simulink model "Elektromagnet_Simscape_Integrated_Model"  (R2025a)
settings: Solver=VariableStepAuto  StartTime=0.0  StopTime=T_sim  RelTol=1e-3
PreLoadFcn:
  | init_simscape_simulation
InitFcn:
  | %init_simscape_simulation
values from neighbouring files (symbols this model uses):
  T_sim = 0.2    [init_simscape_simulation.m]
libraries: fl_lib x8, nesl_utility x6
settings Model: Creator=Polarstern  LastModifiedBy=CelestialAurora

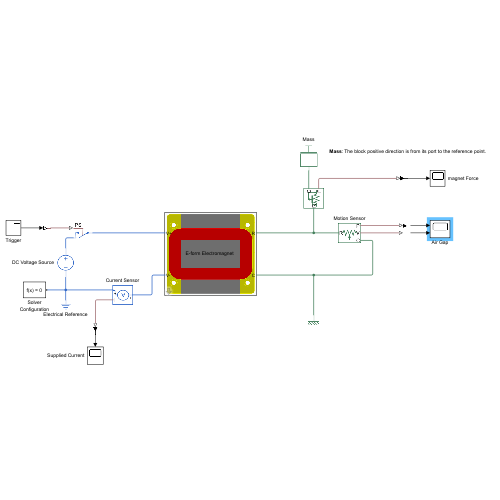
[thumbnail: Simulink's stored preview of the top-level diagram]
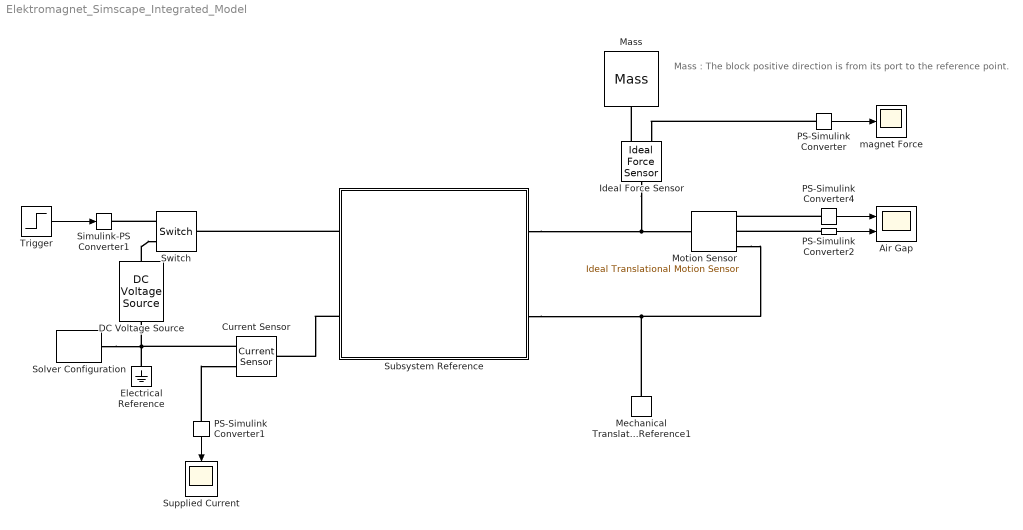
== system Elektromagnet_Simscape_Integrated_Model ==
  note: Mass : The block positive direction is from its port to the reference point.
  Air Gap : Scope  NumInputPorts=2
      settings: Title=Velocity  ActiveDisplayYMinimum=-0.63350040674933106  ActiveDisplayYMaximum=0.42233360449955409
  Current Sensor : fl_lib/Electrical/Electrical Sensors/Current Sensor
  DC Voltage Source : fl_lib/Electrical/Electrical Sources/DC Voltage Source  v0=5 V
  Electrical Reference : fl_lib/Electrical/Electrical Elements/Electrical Reference
  Ideal Force Sensor : fl_lib/Mechanical/Mechanical Sensors/Ideal Force Sensor
  Mass : fl_lib/Mechanical/Translational Elements/Mass  mass=10 kg  num_ports=foundation.enum.numPorts2.one  v_specify=off  v_priority=High  v=0 m/s  v_nominal_specify=off  v_nominal_value=1  v_nominal_unit=m/s  f_specify=off  f_priority=None  f=0 N  f_nominal_specify=on  f_nominal_value=700  f_nominal_unit=N
  Mechanical Translational Reference1 : fl_lib/Mechanical/Translational Elements/Mechanical Translational Reference
  Motion Sensor : fl_lib/Mechanical/Mechanical Sensors/Ideal Translational Motion Sensor  reference=foundation.enum.MeasurementReference.difference  acceleration_port=false  velocity_port=true  position_port=true  offset=airgap_init mm
  PS-Simulink Converter{,1..2,4} (4 alike) : nesl_utility/PS-Simulink Converter  PhysicalDomain=network_engine_domain  SubClassName=ps_output  LeftPortType=input  RightPortType=output  PseudoPeriodic=off  Frequencies=[]  VectorFormat=inherit  Unit=inherit  AffineConversion=off
  Simulink-PS Converter1 : nesl_utility/Simulink-PS Converter  PhysicalDomain=network_engine_domain  SubClassName=ps_input  LeftPortType=input  RightPortType=output  PseudoPeriodic=off  Frequencies=[]  NoiseDistribution=none  NoiseParameters=[]  Unit=1  AffineConversion=off  FilteringAndDerivatives=provide  SimscapeFilterOrder=1  InputFilterTimeConstant=0.001  UdotUserProvided=0
  Solver Configuration : nesl_utility/Solver Configuration  PhysicalDomain=network_engine_domain  SubClassName=solver  LeftPortType=input  RightPortType=generic  Tones=[]  Harmonics=[]  SimulateNoise=off  Profile=off  UseLocalSampling=off  EnableSwitchedLinearOptims=on  FrequencyDomain=off  UseCCode=off  RelTol=0.001  AbsTol=1e-06  MinStep=1e-09  ToWorkspace=off  RevertToSquareIcSolve=off  NumHomotopyIterations=100  PhasorMode=off  PhasorModeNumHarmonics=1  ConsistencySolver=NEWTON_XTOL_AFTER_FTOL  IndexReductionMethod=DerivativeReplacement  DoDC=off  ResidualTolerance=1e-09  ConsistencyTolSource=GLOBAL  ConsistencyAbsTol=0.001  ConsistencyRelTol=0.001  ConsistencyTolFactor=0.001  UseLocalSolver=off  LocalSolverChoice=NE_BACKWARD_EULER_ADVANCER  ResolveIndetEquations=on  FunctionEvalNumThread=1  LocalSolverSampleTime=0.001  DoFixedCost=off  MaxNonlinIter=3  MaxModeIter=2  ComputeImpulses=off  ImpulseIterations=2  LinearAlgebra=auto  LinearAlgebraNumThread=0  EquationFormulation=NE_TIME_EF  DelaysMemoryBudget=1024  AutomaticFiltering=on  FilteringTimeConstant=0.001  PartitionStorageMethod=AS_NEEDED  PartitionMemoryBudget=1024  PartitionMethod=ROBUST  MultibodyUseLocalSolver=off  MultibodyLocalSolverChoice=ODE1  MultibodyLocalSolverSampleTime=0.001
  Subsystem Reference : Subsystem  ReferencedSubsystem=IntegratedElectromagnet  l_airgap=airgap_init
  Supplied Current : Scope
      settings: ActiveDisplayYMinimum=-0.20562097490318823  ActiveDisplayYMaximum=1.8505887741286946  DataLoggingVariableName=ScopeData2
  Switch : fl_lib/Electrical/Electrical Elements/Switch  R_closed=0.01 Ohm  G_open=1e-08 1/Ohm  Threshold=0  i_specify=off  i_priority=High  i=0 A  i_nominal_specify=off  i_nominal_value=1  i_nominal_unit=A  v_specify=off  v_priority=High  v=0 V  v_nominal_specify=off  v_nominal_value=1  v_nominal_unit=V
  Trigger : Step  Time=0.3*T_sim  SampleTime=0
  magnet Force : Scope
      settings: Title=Force  ActiveDisplayYMinimum=-266.85775002835783  ActiveDisplayYMaximum=1052.5296452368557  YLabel=[N]
  wires:
  Trigger/1 -> Simulink-PS Converter1/1
  PS-Simulink Converter1/1 -> Supplied Current/1
  PS-Simulink Converter/1 -> magnet Force/1
  PS-Simulink Converter2/1 -> Air Gap/2
  PS-Simulink Converter4/1 -> Air Gap/1
  connections:
  Current Sensor/RConn2 -- Solver Configuration/RConn1 -- DC Voltage Source/RConn1 -- Electrical Reference/LConn1
  Subsystem Reference/LConn2 -- Current Sensor/LConn1
  Switch/RConn1 -- Simulink-PS Converter1/RConn1
  Subsystem Reference/LConn1 -- Switch/LConn1
  DC Voltage Source/LConn1 -- Switch/RConn2
  PS-Simulink Converter1/LConn1 -- Current Sensor/RConn1
  Ideal Force Sensor/LConn1 -- Subsystem Reference/RConn1 -- Motion Sensor/LConn1
  Motion Sensor/RConn1 -- Subsystem Reference/RConn2 -- Mechanical Translational Reference1/LConn1
  PS-Simulink Converter/LConn1 -- Ideal Force Sensor/RConn2
  PS-Simulink Converter2/LConn1 -- Motion Sensor/RConn2
  PS-Simulink Converter4/LConn1 -- Motion Sensor/RConn3
  Ideal Force Sensor/RConn1 -- Mass/LConn1
